simulink model "test_sys3"  (R2013b)
settings: Solver=ode45  StartTime=0.0  StopTime=5000  RelTol=1e-3
undefined symbols (not defined in the file or in its folder): twiddle_factors
libraries: xbsIndex_r4 x3475, casper_library_misc x231, xps_library x1
(part 1 of 38)
settings Model: Creator=root  LastModifiedBy=root

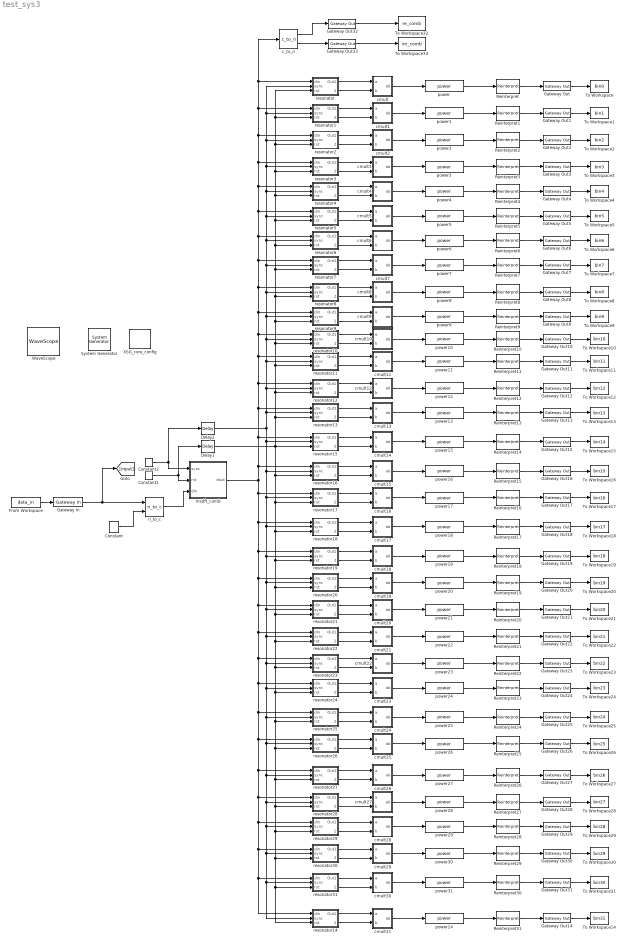
== system test_sys3 ==
  " System Generator" : xbsIndex_r4/ System Generator  Tag=genX  xilinxfamily=Kintex7  part=xc7k325t  speed=-3  package=fbg676  synthesis_tool=XST  clock_wrapper=Clock Enables  directory=./netlist  proj_type=Project Navigator  Synth_file=XST Defaults  Impl_file=ISE Defaults  testbench=off  simulink_period=1  sysclk_period=10  dcm_input_clock_period=10  incr_netlist=off  trim_vbits=Everywhere in SubSystem  dbl_ovrd=According to Block Masks  core_generation=According to Block Masks  run_coregen=off  deprecated_control=off  eval_field=0  block_type=sysgen
  Constant : xbsIndex_r4/Constant  const=0  gui_display_data_type=Fixed-point  arith_type=Signed (2's comp)  n_bits=10  bin_pt=9  preci_type=Single  exp_width=8  frac_width=24  explicit_period=on  period=1  equ=P=C  opselect=C  inp2=PCIN>>17  opr=+  inp1=P  carry=CIN  dbl_ovrd=off  block_type=constant
  Constant1 : xbsIndex_r4/Constant  const=0  gui_display_data_type=Boolean  arith_type=Boolean  n_bits=16  bin_pt=14  preci_type=Single  exp_width=8  frac_width=24  explicit_period=on  period=1  equ=P=C  opselect=C  inp2=PCIN>>17  opr=+  inp1=P  carry=CIN  dbl_ovrd=off  block_type=constant
  Constant2 : xbsIndex_r4/Constant  const=1  gui_display_data_type=Boolean  arith_type=Boolean  n_bits=16  bin_pt=14  preci_type=Single  exp_width=8  frac_width=24  explicit_period=on  period=1  equ=P=C  opselect=C  inp2=PCIN>>17  opr=+  inp1=P  carry=CIN  dbl_ovrd=off  block_type=constant
  Delay1 : xbsIndex_r4/Delay  rst=off  infoeditControl=Selection of Reset will increase slice count due to use of real FFs and instead of SRLs  en=off  latency=1  dbl_ovrd=off  reg_retiming=off  block_type=delay
  Delay2 : xbsIndex_r4/Delay  rst=off  infoeditControl=Selection of Reset will increase slice count due to use of real FFs and instead of SRLs  en=off  latency=1  dbl_ovrd=off  reg_retiming=off  block_type=delay
  From Workspace : FromWorkspace  VariableName=data_in  SampleTime=0
  Gateway In : xbsIndex_r4/Gateway In  gui_display_data_type=Fixed-point  arith_type="Signed  (2's comp)"  n_bits=10  bin_pt=9  preci_type=Single  exp_width=8  frac_width=24  quantization="Round  (unbiased: +/- Inf)"  overflow=Saturate  period=1  dbl_ovrd=off  timing_constraint=None  locs_specified=off  LOCs={}  UseAsADC=off  ADCChannel='1'  inherit_from_input=off  hdl_port=on  block_type=gatewayin
  Gateway Out{,1..33} (34 alike) : xbsIndex_r4/Gateway Out  inherit_from_input=off  hdl_port=on  timing_constraint=None  locs_specified=off  LOCs={}  UseAsDAC=off  DACChannel='1'  block_type=gatewayout
  Reinterpret{,1..31} (32 alike) : xbsIndex_r4/Reinterpret  force_arith_type=off  arith_type=Unsigned  force_bin_pt=on  bin_pt=0  block_type=reinterpret
  To Workspace : ToWorkspace  VariableName=bin0  SampleTime=-1  SaveFormat=Timeseries
  To Workspace1 : ToWorkspace  VariableName=bin1  SampleTime=-1  SaveFormat=Timeseries
  To Workspace10 : ToWorkspace  VariableName=bin10  SampleTime=-1  SaveFormat=Timeseries
  To Workspace11 : ToWorkspace  VariableName=bin11  SampleTime=-1  SaveFormat=Timeseries
  To Workspace12 : ToWorkspace  VariableName=bin12  SampleTime=-1  SaveFormat=Timeseries
  To Workspace13 : ToWorkspace  VariableName=bin13  SampleTime=-1  SaveFormat=Timeseries
  To Workspace14 : ToWorkspace  VariableName=bin31  SampleTime=-1  SaveFormat=Timeseries
  To Workspace15 : ToWorkspace  VariableName=bin14  SampleTime=-1  SaveFormat=Timeseries
  To Workspace16 : ToWorkspace  VariableName=bin15  SampleTime=-1  SaveFormat=Timeseries
  To Workspace17 : ToWorkspace  VariableName=bin16  SampleTime=-1  SaveFormat=Timeseries
  To Workspace18 : ToWorkspace  VariableName=bin17  SampleTime=-1  SaveFormat=Timeseries
  To Workspace19 : ToWorkspace  VariableName=bin18  SampleTime=-1  SaveFormat=Timeseries
  To Workspace2 : ToWorkspace  VariableName=bin2  SampleTime=-1  SaveFormat=Timeseries
  To Workspace20 : ToWorkspace  VariableName=bin19  SampleTime=-1  SaveFormat=Timeseries
  To Workspace21 : ToWorkspace  VariableName=bin20  SampleTime=-1  SaveFormat=Timeseries
  To Workspace22 : ToWorkspace  VariableName=bin21  SampleTime=-1  SaveFormat=Timeseries
  To Workspace23 : ToWorkspace  VariableName=bin22  SampleTime=-1  SaveFormat=Timeseries
  To Workspace24 : ToWorkspace  VariableName=bin23  SampleTime=-1  SaveFormat=Timeseries
  To Workspace25 : ToWorkspace  VariableName=bin24  SampleTime=-1  SaveFormat=Timeseries
  To Workspace26 : ToWorkspace  VariableName=bin25  SampleTime=-1  SaveFormat=Timeseries
  To Workspace27 : ToWorkspace  VariableName=bin26  SampleTime=-1  SaveFormat=Timeseries
  To Workspace28 : ToWorkspace  VariableName=bin27  SampleTime=-1  SaveFormat=Timeseries
  To Workspace29 : ToWorkspace  VariableName=bin28  SampleTime=-1  SaveFormat=Timeseries
  To Workspace3 : ToWorkspace  VariableName=bin3  SampleTime=-1  SaveFormat=Timeseries
  To Workspace30 : ToWorkspace  VariableName=bin29  SampleTime=-1  SaveFormat=Timeseries
  To Workspace31 : ToWorkspace  VariableName=bin30  SampleTime=-1  SaveFormat=Timeseries
  To Workspace32 : ToWorkspace  VariableName=re_comb  SampleTime=-1  SaveFormat=Timeseries
  To Workspace33 : ToWorkspace  VariableName=im_comb  SampleTime=-1  SaveFormat=Timeseries
  To Workspace4 : ToWorkspace  VariableName=bin4  SampleTime=-1  SaveFormat=Timeseries
  To Workspace5 : ToWorkspace  VariableName=bin5  SampleTime=-1  SaveFormat=Timeseries
  To Workspace6 : ToWorkspace  VariableName=bin6  SampleTime=-1  SaveFormat=Timeseries
  To Workspace7 : ToWorkspace  VariableName=bin7  SampleTime=-1  SaveFormat=Timeseries
  To Workspace8 : ToWorkspace  VariableName=bin8  SampleTime=-1  SaveFormat=Timeseries
  To Workspace9 : ToWorkspace  VariableName=bin9  SampleTime=-1  SaveFormat=Timeseries
  WaveScope : xbsIndex_r4/WaveScope  block_type=wavescope
  XSG_core_config : xps_library/XSG_core_config  Tag=xps:xsg  hw_sys=ROACH2:sx475t  clk_src=sys_clk  ROACH_clk_src=sys_clk  ROACH2_clk_src=sys_clk  MKDIG_clk_src=sys_clk  clk_rate=100  sample_period=1  synthesis_tool=XST
  c_to_ri : casper_library_misc/c_to_ri  n_bits=11  bin_pt=9
      settings: AttributesFormatString=11_9 r/i
  cmult : Subsystem  AncestorBlock=casper_library_multipliers/cmult  mask(cmult){n_bits_a=40, bin_pt_a=22, n_bits_b=15, bin_pt_b=13, n_bits_ab=56, bin_pt_ab=35, quantization=Truncate, overflow=Wrap, in_latency=0, mult_latency=3, add_latency=1, conv_latency=1, conjugated=off, async=off, pipelined_enable=on, multiplier_implementation=behavioral HDL}
      mask prompts: n_bits_a "Number of Bits 'a'"; bin_pt_a "Binary Point 'a'"; n_bits_b "Number of Bits 'b'"; bin_pt_b "Binary Point 'b'"; n_bits_ab "Number of Bits 'ab'"; bin_pt_ab "Binary Point 'ab'"; in_latency "Input latency"; mult_latency "Multiplier Latency"; add_latency "Adder Latency"; conv_latency "Convert latency"; conjugated "Conjugate"; async "asynchronous operation"; pipelined_enable "enable pipeline"; multiplier_implementation "Multiplier implementation"
      mask help:
      | Multiplies two complex numbers using 4 multipliers and 2 adders.
      | Conjugation is optional.
      mask init:
      | cmult_init(gcb, ...
      |     'n_bits_a',n_bits_a, ...
      |     'bin_pt_a',bin_pt_a, ...
      |     'n_bits_b',n_bits_b, ...
      |     'bin_pt_b',bin_pt_b, ...
      |     'n_bits_ab',n_bits_ab, ...
      |     'bin_pt_ab',bin_pt_ab, ...
      |     'quantization',quantization, ...
      |     'overflow', overflow, ...
      |     'in_latency', in_latency, ...
      |     'mult_latency', mult_latency, ...
      |     'add_latency', add_latency, ...
      |     'conv_latency', conv_latency, ...
      |     'conjugated', conjugated, ...
      |     'multiplier_implementation', multiplier_implementation, ...
      |     'async', async, ...
      |     'pipelined_enable', pipelined_enable);
      settings: AttributesFormatString=|
      | 40_22 * 15_13 ==> 56_35
      | Truncate, Wrap
      | Latency=0
      mask TypeOptions quantization: Truncate | Round  (unbiased: +/- Inf) | Round  (unbiased: Even Values)
      mask TypeOptions overflow: Wrap | Saturate | Flag as error
      mask TypeOptions multiplier_implementation: behavioral HDL | standard core | embedded multiplier core
  cmult1 : Subsystem  AncestorBlock=casper_library_multipliers/cmult  mask(cmult){n_bits_a=40, bin_pt_a=22, n_bits_b=15, bin_pt_b=13, n_bits_ab=56, bin_pt_ab=35, quantization=Truncate, overflow=Wrap, in_latency=0, mult_latency=3, add_latency=1, conv_latency=1, conjugated=off, async=off, pipelined_enable=on, multiplier_implementation=behavioral HDL}
      mask prompts: n_bits_a "Number of Bits 'a'"; bin_pt_a "Binary Point 'a'"; n_bits_b "Number of Bits 'b'"; bin_pt_b "Binary Point 'b'"; n_bits_ab "Number of Bits 'ab'"; bin_pt_ab "Binary Point 'ab'"; in_latency "Input latency"; mult_latency "Multiplier Latency"; add_latency "Adder Latency"; conv_latency "Convert latency"; conjugated "Conjugate"; async "asynchronous operation"; pipelined_enable "enable pipeline"; multiplier_implementation "Multiplier implementation"
      mask help:
      | Multiplies two complex numbers using 4 multipliers and 2 adders.
      | Conjugation is optional.
      mask init: same as test_sys3/cmult
      settings: AttributesFormatString=|
      | 40_22 * 15_13 ==> 56_35
      | Truncate, Wrap
      | Latency=0
      mask TypeOptions quantization: Truncate | Round  (unbiased: +/- Inf) | Round  (unbiased: Even Values)
      mask TypeOptions overflow: Wrap | Saturate | Flag as error
      mask TypeOptions multiplier_implementation: behavioral HDL | standard core | embedded multiplier core
  cmult10 : Subsystem  AncestorBlock=casper_library_multipliers/cmult  mask(cmult){n_bits_a=40, bin_pt_a=22, n_bits_b=15, bin_pt_b=13, n_bits_ab=56, bin_pt_ab=35, quantization=Truncate, overflow=Wrap, in_latency=0, mult_latency=3, add_latency=1, conv_latency=1, conjugated=off, async=off, pipelined_enable=on, multiplier_implementation=behavioral HDL}
      mask prompts: n_bits_a "Number of Bits 'a'"; bin_pt_a "Binary Point 'a'"; n_bits_b "Number of Bits 'b'"; bin_pt_b "Binary Point 'b'"; n_bits_ab "Number of Bits 'ab'"; bin_pt_ab "Binary Point 'ab'"; in_latency "Input latency"; mult_latency "Multiplier Latency"; add_latency "Adder Latency"; conv_latency "Convert latency"; conjugated "Conjugate"; async "asynchronous operation"; pipelined_enable "enable pipeline"; multiplier_implementation "Multiplier implementation"
      mask help:
      | Multiplies two complex numbers using 4 multipliers and 2 adders.
      | Conjugation is optional.
      mask init: same as test_sys3/cmult
      settings: AttributesFormatString=|
      | 40_22 * 15_13 ==> 56_35
      | Truncate, Wrap
      | Latency=0
      mask TypeOptions quantization: Truncate | Round  (unbiased: +/- Inf) | Round  (unbiased: Even Values)
      mask TypeOptions overflow: Wrap | Saturate | Flag as error
      mask TypeOptions multiplier_implementation: behavioral HDL | standard core | embedded multiplier core
  cmult11 : Subsystem  AncestorBlock=casper_library_multipliers/cmult  mask(cmult){n_bits_a=40, bin_pt_a=22, n_bits_b=15, bin_pt_b=13, n_bits_ab=56, bin_pt_ab=35, quantization=Truncate, overflow=Wrap, in_latency=0, mult_latency=3, add_latency=1, conv_latency=1, conjugated=off, async=off, pipelined_enable=on, multiplier_implementation=behavioral HDL}
      mask prompts: n_bits_a "Number of Bits 'a'"; bin_pt_a "Binary Point 'a'"; n_bits_b "Number of Bits 'b'"; bin_pt_b "Binary Point 'b'"; n_bits_ab "Number of Bits 'ab'"; bin_pt_ab "Binary Point 'ab'"; in_latency "Input latency"; mult_latency "Multiplier Latency"; add_latency "Adder Latency"; conv_latency "Convert latency"; conjugated "Conjugate"; async "asynchronous operation"; pipelined_enable "enable pipeline"; multiplier_implementation "Multiplier implementation"
      mask help:
      | Multiplies two complex numbers using 4 multipliers and 2 adders.
      | Conjugation is optional.
      mask init: same as test_sys3/cmult
      settings: AttributesFormatString=|
      | 40_22 * 15_13 ==> 56_35
      | Truncate, Wrap
      | Latency=0
      mask TypeOptions quantization: Truncate | Round  (unbiased: +/- Inf) | Round  (unbiased: Even Values)
      mask TypeOptions overflow: Wrap | Saturate | Flag as error
      mask TypeOptions multiplier_implementation: behavioral HDL | standard core | embedded multiplier core
  cmult12 : Subsystem  AncestorBlock=casper_library_multipliers/cmult  mask(cmult){n_bits_a=40, bin_pt_a=22, n_bits_b=15, bin_pt_b=13, n_bits_ab=56, bin_pt_ab=35, quantization=Truncate, overflow=Wrap, in_latency=0, mult_latency=3, add_latency=1, conv_latency=1, conjugated=off, async=off, pipelined_enable=on, multiplier_implementation=behavioral HDL}
      mask prompts: n_bits_a "Number of Bits 'a'"; bin_pt_a "Binary Point 'a'"; n_bits_b "Number of Bits 'b'"; bin_pt_b "Binary Point 'b'"; n_bits_ab "Number of Bits 'ab'"; bin_pt_ab "Binary Point 'ab'"; in_latency "Input latency"; mult_latency "Multiplier Latency"; add_latency "Adder Latency"; conv_latency "Convert latency"; conjugated "Conjugate"; async "asynchronous operation"; pipelined_enable "enable pipeline"; multiplier_implementation "Multiplier implementation"
      mask help:
      | Multiplies two complex numbers using 4 multipliers and 2 adders.
      | Conjugation is optional.
      mask init: same as test_sys3/cmult
      settings: AttributesFormatString=|
      | 40_22 * 15_13 ==> 56_35
      | Truncate, Wrap
      | Latency=0
      mask TypeOptions quantization: Truncate | Round  (unbiased: +/- Inf) | Round  (unbiased: Even Values)
      mask TypeOptions overflow: Wrap | Saturate | Flag as error
      mask TypeOptions multiplier_implementation: behavioral HDL | standard core | embedded multiplier core
  cmult13 : Subsystem  AncestorBlock=casper_library_multipliers/cmult  mask(cmult){n_bits_a=40, bin_pt_a=22, n_bits_b=15, bin_pt_b=13, n_bits_ab=56, bin_pt_ab=35, quantization=Truncate, overflow=Wrap, in_latency=0, mult_latency=3, add_latency=1, conv_latency=1, conjugated=off, async=off, pipelined_enable=on, multiplier_implementation=behavioral HDL}
      mask prompts: n_bits_a "Number of Bits 'a'"; bin_pt_a "Binary Point 'a'"; n_bits_b "Number of Bits 'b'"; bin_pt_b "Binary Point 'b'"; n_bits_ab "Number of Bits 'ab'"; bin_pt_ab "Binary Point 'ab'"; in_latency "Input latency"; mult_latency "Multiplier Latency"; add_latency "Adder Latency"; conv_latency "Convert latency"; conjugated "Conjugate"; async "asynchronous operation"; pipelined_enable "enable pipeline"; multiplier_implementation "Multiplier implementation"
      mask help:
      | Multiplies two complex numbers using 4 multipliers and 2 adders.
      | Conjugation is optional.
      mask init: same as test_sys3/cmult
      settings: AttributesFormatString=|
      | 40_22 * 15_13 ==> 56_35
      | Truncate, Wrap
      | Latency=0
      mask TypeOptions quantization: Truncate | Round  (unbiased: +/- Inf) | Round  (unbiased: Even Values)
      mask TypeOptions overflow: Wrap | Saturate | Flag as error
      mask TypeOptions multiplier_implementation: behavioral HDL | standard core | embedded multiplier core
  cmult14 : Subsystem  AncestorBlock=casper_library_multipliers/cmult  mask(cmult){n_bits_a=40, bin_pt_a=22, n_bits_b=15, bin_pt_b=13, n_bits_ab=56, bin_pt_ab=35, quantization=Truncate, overflow=Wrap, in_latency=0, mult_latency=3, add_latency=1, conv_latency=1, conjugated=off, async=off, pipelined_enable=on, multiplier_implementation=behavioral HDL}
      mask prompts: n_bits_a "Number of Bits 'a'"; bin_pt_a "Binary Point 'a'"; n_bits_b "Number of Bits 'b'"; bin_pt_b "Binary Point 'b'"; n_bits_ab "Number of Bits 'ab'"; bin_pt_ab "Binary Point 'ab'"; in_latency "Input latency"; mult_latency "Multiplier Latency"; add_latency "Adder Latency"; conv_latency "Convert latency"; conjugated "Conjugate"; async "asynchronous operation"; pipelined_enable "enable pipeline"; multiplier_implementation "Multiplier implementation"
      mask help:
      | Multiplies two complex numbers using 4 multipliers and 2 adders.
      | Conjugation is optional.
      mask init: same as test_sys3/cmult
      settings: AttributesFormatString=|
      | 40_22 * 15_13 ==> 56_35
      | Truncate, Wrap
      | Latency=0
      mask TypeOptions quantization: Truncate | Round  (unbiased: +/- Inf) | Round  (unbiased: Even Values)
      mask TypeOptions overflow: Wrap | Saturate | Flag as error
      mask TypeOptions multiplier_implementation: behavioral HDL | standard core | embedded multiplier core
  cmult15 : Subsystem  AncestorBlock=casper_library_multipliers/cmult  mask(cmult){n_bits_a=40, bin_pt_a=22, n_bits_b=15, bin_pt_b=13, n_bits_ab=56, bin_pt_ab=35, quantization=Truncate, overflow=Wrap, in_latency=0, mult_latency=3, add_latency=1, conv_latency=1, conjugated=off, async=off, pipelined_enable=on, multiplier_implementation=behavioral HDL}
      mask prompts: n_bits_a "Number of Bits 'a'"; bin_pt_a "Binary Point 'a'"; n_bits_b "Number of Bits 'b'"; bin_pt_b "Binary Point 'b'"; n_bits_ab "Number of Bits 'ab'"; bin_pt_ab "Binary Point 'ab'"; in_latency "Input latency"; mult_latency "Multiplier Latency"; add_latency "Adder Latency"; conv_latency "Convert latency"; conjugated "Conjugate"; async "asynchronous operation"; pipelined_enable "enable pipeline"; multiplier_implementation "Multiplier implementation"
      mask help:
      | Multiplies two complex numbers using 4 multipliers and 2 adders.
      | Conjugation is optional.
      mask init: same as test_sys3/cmult
      settings: AttributesFormatString=|
      | 40_22 * 15_13 ==> 56_35
      | Truncate, Wrap
      | Latency=0
      mask TypeOptions quantization: Truncate | Round  (unbiased: +/- Inf) | Round  (unbiased: Even Values)
      mask TypeOptions overflow: Wrap | Saturate | Flag as error
      mask TypeOptions multiplier_implementation: behavioral HDL | standard core | embedded multiplier core
  cmult16 : Subsystem  AncestorBlock=casper_library_multipliers/cmult  mask(cmult){n_bits_a=40, bin_pt_a=22, n_bits_b=15, bin_pt_b=13, n_bits_ab=56, bin_pt_ab=35, quantization=Truncate, overflow=Wrap, in_latency=0, mult_latency=3, add_latency=1, conv_latency=1, conjugated=off, async=off, pipelined_enable=on, multiplier_implementation=behavioral HDL}
      mask prompts: n_bits_a "Number of Bits 'a'"; bin_pt_a "Binary Point 'a'"; n_bits_b "Number of Bits 'b'"; bin_pt_b "Binary Point 'b'"; n_bits_ab "Number of Bits 'ab'"; bin_pt_ab "Binary Point 'ab'"; in_latency "Input latency"; mult_latency "Multiplier Latency"; add_latency "Adder Latency"; conv_latency "Convert latency"; conjugated "Conjugate"; async "asynchronous operation"; pipelined_enable "enable pipeline"; multiplier_implementation "Multiplier implementation"
      mask help:
      | Multiplies two complex numbers using 4 multipliers and 2 adders.
      | Conjugation is optional.
      mask init: same as test_sys3/cmult
      settings: AttributesFormatString=|
      | 40_22 * 15_13 ==> 56_35
      | Truncate, Wrap
      | Latency=0
      mask TypeOptions quantization: Truncate | Round  (unbiased: +/- Inf) | Round  (unbiased: Even Values)
      mask TypeOptions overflow: Wrap | Saturate | Flag as error
      mask TypeOptions multiplier_implementation: behavioral HDL | standard core | embedded multiplier core
  cmult17 : Subsystem  AncestorBlock=casper_library_multipliers/cmult  mask(cmult){n_bits_a=40, bin_pt_a=22, n_bits_b=15, bin_pt_b=13, n_bits_ab=56, bin_pt_ab=35, quantization=Truncate, overflow=Wrap, in_latency=0, mult_latency=3, add_latency=1, conv_latency=1, conjugated=off, async=off, pipelined_enable=on, multiplier_implementation=behavioral HDL}
      mask prompts: n_bits_a "Number of Bits 'a'"; bin_pt_a "Binary Point 'a'"; n_bits_b "Number of Bits 'b'"; bin_pt_b "Binary Point 'b'"; n_bits_ab "Number of Bits 'ab'"; bin_pt_ab "Binary Point 'ab'"; in_latency "Input latency"; mult_latency "Multiplier Latency"; add_latency "Adder Latency"; conv_latency "Convert latency"; conjugated "Conjugate"; async "asynchronous operation"; pipelined_enable "enable pipeline"; multiplier_implementation "Multiplier implementation"
      mask help:
      | Multiplies two complex numbers using 4 multipliers and 2 adders.
      | Conjugation is optional.
      mask init: same as test_sys3/cmult
      settings: AttributesFormatString=|
      | 40_22 * 15_13 ==> 56_35
      | Truncate, Wrap
      | Latency=0
      mask TypeOptions quantization: Truncate | Round  (unbiased: +/- Inf) | Round  (unbiased: Even Values)
      mask TypeOptions overflow: Wrap | Saturate | Flag as error
      mask TypeOptions multiplier_implementation: behavioral HDL | standard core | embedded multiplier core
  cmult18 : Subsystem  AncestorBlock=casper_library_multipliers/cmult  mask(cmult){n_bits_a=40, bin_pt_a=22, n_bits_b=15, bin_pt_b=13, n_bits_ab=56, bin_pt_ab=35, quantization=Truncate, overflow=Wrap, in_latency=0, mult_latency=3, add_latency=1, conv_latency=1, conjugated=off, async=off, pipelined_enable=on, multiplier_implementation=behavioral HDL}
      mask prompts: n_bits_a "Number of Bits 'a'"; bin_pt_a "Binary Point 'a'"; n_bits_b "Number of Bits 'b'"; bin_pt_b "Binary Point 'b'"; n_bits_ab "Number of Bits 'ab'"; bin_pt_ab "Binary Point 'ab'"; in_latency "Input latency"; mult_latency "Multiplier Latency"; add_latency "Adder Latency"; conv_latency "Convert latency"; conjugated "Conjugate"; async "asynchronous operation"; pipelined_enable "enable pipeline"; multiplier_implementation "Multiplier implementation"
      mask help:
      | Multiplies two complex numbers using 4 multipliers and 2 adders.
      | Conjugation is optional.
      mask init: same as test_sys3/cmult
      settings: AttributesFormatString=|
      | 40_22 * 15_13 ==> 56_35
      | Truncate, Wrap
      | Latency=0
      mask TypeOptions quantization: Truncate | Round  (unbiased: +/- Inf) | Round  (unbiased: Even Values)
      mask TypeOptions overflow: Wrap | Saturate | Flag as error
      mask TypeOptions multiplier_implementation: behavioral HDL | standard core | embedded multiplier core
  cmult19 : Subsystem  AncestorBlock=casper_library_multipliers/cmult  mask(cmult){n_bits_a=40, bin_pt_a=22, n_bits_b=15, bin_pt_b=13, n_bits_ab=56, bin_pt_ab=35, quantization=Truncate, overflow=Wrap, in_latency=0, mult_latency=3, add_latency=1, conv_latency=1, conjugated=off, async=off, pipelined_enable=on, multiplier_implementation=behavioral HDL}
      mask prompts: n_bits_a "Number of Bits 'a'"; bin_pt_a "Binary Point 'a'"; n_bits_b "Number of Bits 'b'"; bin_pt_b "Binary Point 'b'"; n_bits_ab "Number of Bits 'ab'"; bin_pt_ab "Binary Point 'ab'"; in_latency "Input latency"; mult_latency "Multiplier Latency"; add_latency "Adder Latency"; conv_latency "Convert latency"; conjugated "Conjugate"; async "asynchronous operation"; pipelined_enable "enable pipeline"; multiplier_implementation "Multiplier implementation"
      mask help:
      | Multiplies two complex numbers using 4 multipliers and 2 adders.
      | Conjugation is optional.
      mask init: same as test_sys3/cmult
      settings: AttributesFormatString=|
      | 40_22 * 15_13 ==> 56_35
      | Truncate, Wrap
      | Latency=0
      mask TypeOptions quantization: Truncate | Round  (unbiased: +/- Inf) | Round  (unbiased: Even Values)
      mask TypeOptions overflow: Wrap | Saturate | Flag as error
      mask TypeOptions multiplier_implementation: behavioral HDL | standard core | embedded multiplier core
  cmult2 : Subsystem  AncestorBlock=casper_library_multipliers/cmult  mask(cmult){n_bits_a=40, bin_pt_a=22, n_bits_b=15, bin_pt_b=13, n_bits_ab=56, bin_pt_ab=35, quantization=Truncate, overflow=Wrap, in_latency=0, mult_latency=3, add_latency=1, conv_latency=1, conjugated=off, async=off, pipelined_enable=on, multiplier_implementation=behavioral HDL}
      mask prompts: n_bits_a "Number of Bits 'a'"; bin_pt_a "Binary Point 'a'"; n_bits_b "Number of Bits 'b'"; bin_pt_b "Binary Point 'b'"; n_bits_ab "Number of Bits 'ab'"; bin_pt_ab "Binary Point 'ab'"; in_latency "Input latency"; mult_latency "Multiplier Latency"; add_latency "Adder Latency"; conv_latency "Convert latency"; conjugated "Conjugate"; async "asynchronous operation"; pipelined_enable "enable pipeline"; multiplier_implementation "Multiplier implementation"
      mask help:
      | Multiplies two complex numbers using 4 multipliers and 2 adders.
      | Conjugation is optional.
      mask init: same as test_sys3/cmult
      settings: AttributesFormatString=|
      | 40_22 * 15_13 ==> 56_35
      | Truncate, Wrap
      | Latency=0
      mask TypeOptions quantization: Truncate | Round  (unbiased: +/- Inf) | Round  (unbiased: Even Values)
      mask TypeOptions overflow: Wrap | Saturate | Flag as error
      mask TypeOptions multiplier_implementation: behavioral HDL | standard core | embedded multiplier core
  cmult20 : Subsystem  AncestorBlock=casper_library_multipliers/cmult  mask(cmult){n_bits_a=40, bin_pt_a=22, n_bits_b=15, bin_pt_b=13, n_bits_ab=56, bin_pt_ab=35, quantization=Truncate, overflow=Wrap, in_latency=0, mult_latency=3, add_latency=1, conv_latency=1, conjugated=off, async=off, pipelined_enable=on, multiplier_implementation=behavioral HDL}
      mask prompts: n_bits_a "Number of Bits 'a'"; bin_pt_a "Binary Point 'a'"; n_bits_b "Number of Bits 'b'"; bin_pt_b "Binary Point 'b'"; n_bits_ab "Number of Bits 'ab'"; bin_pt_ab "Binary Point 'ab'"; in_latency "Input latency"; mult_latency "Multiplier Latency"; add_latency "Adder Latency"; conv_latency "Convert latency"; conjugated "Conjugate"; async "asynchronous operation"; pipelined_enable "enable pipeline"; multiplier_implementation "Multiplier implementation"
      mask help:
      | Multiplies two complex numbers using 4 multipliers and 2 adders.
      | Conjugation is optional.
      mask init: same as test_sys3/cmult
      settings: AttributesFormatString=|
      | 40_22 * 15_13 ==> 56_35
      | Truncate, Wrap
      | Latency=0
      mask TypeOptions quantization: Truncate | Round  (unbiased: +/- Inf) | Round  (unbiased: Even Values)
      mask TypeOptions overflow: Wrap | Saturate | Flag as error
      mask TypeOptions multiplier_implementation: behavioral HDL | standard core | embedded multiplier core
  cmult21 : Subsystem  AncestorBlock=casper_library_multipliers/cmult  mask(cmult){n_bits_a=40, bin_pt_a=22, n_bits_b=15, bin_pt_b=13, n_bits_ab=56, bin_pt_ab=35, quantization=Truncate, overflow=Wrap, in_latency=0, mult_latency=3, add_latency=1, conv_latency=1, conjugated=off, async=off, pipelined_enable=on, multiplier_implementation=behavioral HDL}
      mask prompts: n_bits_a "Number of Bits 'a'"; bin_pt_a "Binary Point 'a'"; n_bits_b "Number of Bits 'b'"; bin_pt_b "Binary Point 'b'"; n_bits_ab "Number of Bits 'ab'"; bin_pt_ab "Binary Point 'ab'"; in_latency "Input latency"; mult_latency "Multiplier Latency"; add_latency "Adder Latency"; conv_latency "Convert latency"; conjugated "Conjugate"; async "asynchronous operation"; pipelined_enable "enable pipeline"; multiplier_implementation "Multiplier implementation"
      mask help:
      | Multiplies two complex numbers using 4 multipliers and 2 adders.
      | Conjugation is optional.
      mask init: same as test_sys3/cmult
      settings: AttributesFormatString=|
      | 40_22 * 15_13 ==> 56_35
      | Truncate, Wrap
      | Latency=0
      mask TypeOptions quantization: Truncate | Round  (unbiased: +/- Inf) | Round  (unbiased: Even Values)
      mask TypeOptions overflow: Wrap | Saturate | Flag as error
      mask TypeOptions multiplier_implementation: behavioral HDL | standard core | embedded multiplier core
  cmult22 : Subsystem  AncestorBlock=casper_library_multipliers/cmult  mask(cmult){n_bits_a=40, bin_pt_a=22, n_bits_b=15, bin_pt_b=13, n_bits_ab=56, bin_pt_ab=35, quantization=Truncate, overflow=Wrap, in_latency=0, mult_latency=3, add_latency=1, conv_latency=1, conjugated=off, async=off, pipelined_enable=on, multiplier_implementation=behavioral HDL}
      mask prompts: n_bits_a "Number of Bits 'a'"; bin_pt_a "Binary Point 'a'"; n_bits_b "Number of Bits 'b'"; bin_pt_b "Binary Point 'b'"; n_bits_ab "Number of Bits 'ab'"; bin_pt_ab "Binary Point 'ab'"; in_latency "Input latency"; mult_latency "Multiplier Latency"; add_latency "Adder Latency"; conv_latency "Convert latency"; conjugated "Conjugate"; async "asynchronous operation"; pipelined_enable "enable pipeline"; multiplier_implementation "Multiplier implementation"
      mask help:
      | Multiplies two complex numbers using 4 multipliers and 2 adders.
      | Conjugation is optional.
      mask init: same as test_sys3/cmult
      settings: AttributesFormatString=|
      | 40_22 * 15_13 ==> 56_35
      | Truncate, Wrap
      | Latency=0
      mask TypeOptions quantization: Truncate | Round  (unbiased: +/- Inf) | Round  (unbiased: Even Values)
      mask TypeOptions overflow: Wrap | Saturate | Flag as error
      mask TypeOptions multiplier_implementation: behavioral HDL | standard core | embedded multiplier core
  cmult23 : Subsystem  AncestorBlock=casper_library_multipliers/cmult  mask(cmult){n_bits_a=40, bin_pt_a=22, n_bits_b=15, bin_pt_b=13, n_bits_ab=56, bin_pt_ab=35, quantization=Truncate, overflow=Wrap, in_latency=0, mult_latency=3, add_latency=1, conv_latency=1, conjugated=off, async=off, pipelined_enable=on, multiplier_implementation=behavioral HDL}
      mask prompts: n_bits_a "Number of Bits 'a'"; bin_pt_a "Binary Point 'a'"; n_bits_b "Number of Bits 'b'"; bin_pt_b "Binary Point 'b'"; n_bits_ab "Number of Bits 'ab'"; bin_pt_ab "Binary Point 'ab'"; in_latency "Input latency"; mult_latency "Multiplier Latency"; add_latency "Adder Latency"; conv_latency "Convert latency"; conjugated "Conjugate"; async "asynchronous operation"; pipelined_enable "enable pipeline"; multiplier_implementation "Multiplier implementation"
      mask help:
      | Multiplies two complex numbers using 4 multipliers and 2 adders.
      | Conjugation is optional.
      mask init: same as test_sys3/cmult
      settings: AttributesFormatString=|
      | 40_22 * 15_13 ==> 56_35
      | Truncate, Wrap
      | Latency=0
      mask TypeOptions quantization: Truncate | Round  (unbiased: +/- Inf) | Round  (unbiased: Even Values)
      mask TypeOptions overflow: Wrap | Saturate | Flag as error
      mask TypeOptions multiplier_implementation: behavioral HDL | standard core | embedded multiplier core
  cmult24 : Subsystem  AncestorBlock=casper_library_multipliers/cmult  mask(cmult){n_bits_a=40, bin_pt_a=22, n_bits_b=15, bin_pt_b=13, n_bits_ab=56, bin_pt_ab=35, quantization=Truncate, overflow=Wrap, in_latency=0, mult_latency=3, add_latency=1, conv_latency=1, conjugated=off, async=off, pipelined_enable=on, multiplier_implementation=behavioral HDL}
      mask prompts: n_bits_a "Number of Bits 'a'"; bin_pt_a "Binary Point 'a'"; n_bits_b "Number of Bits 'b'"; bin_pt_b "Binary Point 'b'"; n_bits_ab "Number of Bits 'ab'"; bin_pt_ab "Binary Point 'ab'"; in_latency "Input latency"; mult_latency "Multiplier Latency"; add_latency "Adder Latency"; conv_latency "Convert latency"; conjugated "Conjugate"; async "asynchronous operation"; pipelined_enable "enable pipeline"; multiplier_implementation "Multiplier implementation"
      mask help:
      | Multiplies two complex numbers using 4 multipliers and 2 adders.
      | Conjugation is optional.
      mask init: same as test_sys3/cmult
      settings: AttributesFormatString=|
      | 40_22 * 15_13 ==> 56_35
      | Truncate, Wrap
      | Latency=0
      mask TypeOptions quantization: Truncate | Round  (unbiased: +/- Inf) | Round  (unbiased: Even Values)
      mask TypeOptions overflow: Wrap | Saturate | Flag as error
      mask TypeOptions multiplier_implementation: behavioral HDL | standard core | embedded multiplier core
  cmult25 : Subsystem  AncestorBlock=casper_library_multipliers/cmult  mask(cmult){n_bits_a=40, bin_pt_a=22, n_bits_b=15, bin_pt_b=13, n_bits_ab=56, bin_pt_ab=35, quantization=Truncate, overflow=Wrap, in_latency=0, mult_latency=3, add_latency=1, conv_latency=1, conjugated=off, async=off, pipelined_enable=on, multiplier_implementation=behavioral HDL}
      mask prompts: n_bits_a "Number of Bits 'a'"; bin_pt_a "Binary Point 'a'"; n_bits_b "Number of Bits 'b'"; bin_pt_b "Binary Point 'b'"; n_bits_ab "Number of Bits 'ab'"; bin_pt_ab "Binary Point 'ab'"; in_latency "Input latency"; mult_latency "Multiplier Latency"; add_latency "Adder Latency"; conv_latency "Convert latency"; conjugated "Conjugate"; async "asynchronous operation"; pipelined_enable "enable pipeline"; multiplier_implementation "Multiplier implementation"
      mask help:
      | Multiplies two complex numbers using 4 multipliers and 2 adders.
      | Conjugation is optional.
      mask init: same as test_sys3/cmult
      settings: AttributesFormatString=|
      | 40_22 * 15_13 ==> 56_35
      | Truncate, Wrap
      | Latency=0
      mask TypeOptions quantization: Truncate | Round  (unbiased: +/- Inf) | Round  (unbiased: Even Values)
      mask TypeOptions overflow: Wrap | Saturate | Flag as error
      mask TypeOptions multiplier_implementation: behavioral HDL | standard core | embedded multiplier core
  cmult26 : Subsystem  AncestorBlock=casper_library_multipliers/cmult  mask(cmult){n_bits_a=40, bin_pt_a=22, n_bits_b=15, bin_pt_b=13, n_bits_ab=56, bin_pt_ab=35, quantization=Truncate, overflow=Wrap, in_latency=0, mult_latency=3, add_latency=1, conv_latency=1, conjugated=off, async=off, pipelined_enable=on, multiplier_implementation=behavioral HDL}
      mask prompts: n_bits_a "Number of Bits 'a'"; bin_pt_a "Binary Point 'a'"; n_bits_b "Number of Bits 'b'"; bin_pt_b "Binary Point 'b'"; n_bits_ab "Number of Bits 'ab'"; bin_pt_ab "Binary Point 'ab'"; in_latency "Input latency"; mult_latency "Multiplier Latency"; add_latency "Adder Latency"; conv_latency "Convert latency"; conjugated "Conjugate"; async "asynchronous operation"; pipelined_enable "enable pipeline"; multiplier_implementation "Multiplier implementation"
      mask help:
      | Multiplies two complex numbers using 4 multipliers and 2 adders.
      | Conjugation is optional.
      mask init: same as test_sys3/cmult
      settings: AttributesFormatString=|
      | 40_22 * 15_13 ==> 56_35
      | Truncate, Wrap
      | Latency=0
      mask TypeOptions quantization: Truncate | Round  (unbiased: +/- Inf) | Round  (unbiased: Even Values)
      mask TypeOptions overflow: Wrap | Saturate | Flag as error
      mask TypeOptions multiplier_implementation: behavioral HDL | standard core | embedded multiplier core
  cmult27 : Subsystem  AncestorBlock=casper_library_multipliers/cmult  mask(cmult){n_bits_a=40, bin_pt_a=22, n_bits_b=15, bin_pt_b=13, n_bits_ab=56, bin_pt_ab=35, quantization=Truncate, overflow=Wrap, in_latency=0, mult_latency=3, add_latency=1, conv_latency=1, conjugated=off, async=off, pipelined_enable=on, multiplier_implementation=behavioral HDL}
      mask prompts: n_bits_a "Number of Bits 'a'"; bin_pt_a "Binary Point 'a'"; n_bits_b "Number of Bits 'b'"; bin_pt_b "Binary Point 'b'"; n_bits_ab "Number of Bits 'ab'"; bin_pt_ab "Binary Point 'ab'"; in_latency "Input latency"; mult_latency "Multiplier Latency"; add_latency "Adder Latency"; conv_latency "Convert latency"; conjugated "Conjugate"; async "asynchronous operation"; pipelined_enable "enable pipeline"; multiplier_implementation "Multiplier implementation"
      mask help:
      | Multiplies two complex numbers using 4 multipliers and 2 adders.
      | Conjugation is optional.
      mask init: same as test_sys3/cmult
      settings: AttributesFormatString=|
      | 40_22 * 15_13 ==> 56_35
      | Truncate, Wrap
      | Latency=0
      mask TypeOptions quantization: Truncate | Round  (unbiased: +/- Inf) | Round  (unbiased: Even Values)
      mask TypeOptions overflow: Wrap | Saturate | Flag as error
      mask TypeOptions multiplier_implementation: behavioral HDL | standard core | embedded multiplier core
  cmult28 : Subsystem  AncestorBlock=casper_library_multipliers/cmult  mask(cmult){n_bits_a=40, bin_pt_a=22, n_bits_b=15, bin_pt_b=13, n_bits_ab=56, bin_pt_ab=35, quantization=Truncate, overflow=Wrap, in_latency=0, mult_latency=3, add_latency=1, conv_latency=1, conjugated=off, async=off, pipelined_enable=on, multiplier_implementation=behavioral HDL}
      mask prompts: n_bits_a "Number of Bits 'a'"; bin_pt_a "Binary Point 'a'"; n_bits_b "Number of Bits 'b'"; bin_pt_b "Binary Point 'b'"; n_bits_ab "Number of Bits 'ab'"; bin_pt_ab "Binary Point 'ab'"; in_latency "Input latency"; mult_latency "Multiplier Latency"; add_latency "Adder Latency"; conv_latency "Convert latency"; conjugated "Conjugate"; async "asynchronous operation"; pipelined_enable "enable pipeline"; multiplier_implementation "Multiplier implementation"
      mask help:
      | Multiplies two complex numbers using 4 multipliers and 2 adders.
      | Conjugation is optional.
      mask init: same as test_sys3/cmult
      settings: AttributesFormatString=|
      | 40_22 * 15_13 ==> 56_35
      | Truncate, Wrap
      | Latency=0
      mask TypeOptions quantization: Truncate | Round  (unbiased: +/- Inf) | Round  (unbiased: Even Values)
      mask TypeOptions overflow: Wrap | Saturate | Flag as error
      mask TypeOptions multiplier_implementation: behavioral HDL | standard core | embedded multiplier core
  cmult29 : Subsystem  AncestorBlock=casper_library_multipliers/cmult  mask(cmult){n_bits_a=40, bin_pt_a=22, n_bits_b=15, bin_pt_b=13, n_bits_ab=56, bin_pt_ab=35, quantization=Truncate, overflow=Wrap, in_latency=0, mult_latency=3, add_latency=1, conv_latency=1, conjugated=off, async=off, pipelined_enable=on, multiplier_implementation=behavioral HDL}
      mask prompts: n_bits_a "Number of Bits 'a'"; bin_pt_a "Binary Point 'a'"; n_bits_b "Number of Bits 'b'"; bin_pt_b "Binary Point 'b'"; n_bits_ab "Number of Bits 'ab'"; bin_pt_ab "Binary Point 'ab'"; in_latency "Input latency"; mult_latency "Multiplier Latency"; add_latency "Adder Latency"; conv_latency "Convert latency"; conjugated "Conjugate"; async "asynchronous operation"; pipelined_enable "enable pipeline"; multiplier_implementation "Multiplier implementation"
      mask help:
      | Multiplies two complex numbers using 4 multipliers and 2 adders.
      | Conjugation is optional.
      mask init: same as test_sys3/cmult
      settings: AttributesFormatString=|
      | 40_22 * 15_13 ==> 56_35
      | Truncate, Wrap
      | Latency=0
      mask TypeOptions quantization: Truncate | Round  (unbiased: +/- Inf) | Round  (unbiased: Even Values)
      mask TypeOptions overflow: Wrap | Saturate | Flag as error
      mask TypeOptions multiplier_implementation: behavioral HDL | standard core | embedded multiplier core
  cmult3 : Subsystem  AncestorBlock=casper_library_multipliers/cmult  mask(cmult){n_bits_a=40, bin_pt_a=22, n_bits_b=15, bin_pt_b=13, n_bits_ab=56, bin_pt_ab=35, quantization=Truncate, overflow=Wrap, in_latency=0, mult_latency=3, add_latency=1, conv_latency=1, conjugated=off, async=off, pipelined_enable=on, multiplier_implementation=behavioral HDL}
      mask prompts: n_bits_a "Number of Bits 'a'"; bin_pt_a "Binary Point 'a'"; n_bits_b "Number of Bits 'b'"; bin_pt_b "Binary Point 'b'"; n_bits_ab "Number of Bits 'ab'"; bin_pt_ab "Binary Point 'ab'"; in_latency "Input latency"; mult_latency "Multiplier Latency"; add_latency "Adder Latency"; conv_latency "Convert latency"; conjugated "Conjugate"; async "asynchronous operation"; pipelined_enable "enable pipeline"; multiplier_implementation "Multiplier implementation"
      mask help:
      | Multiplies two complex numbers using 4 multipliers and 2 adders.
      | Conjugation is optional.
      mask init: same as test_sys3/cmult
      settings: AttributesFormatString=|
      | 40_22 * 15_13 ==> 56_35
      | Truncate, Wrap
      | Latency=0
      mask TypeOptions quantization: Truncate | Round  (unbiased: +/- Inf) | Round  (unbiased: Even Values)
      mask TypeOptions overflow: Wrap | Saturate | Flag as error
      mask TypeOptions multiplier_implementation: behavioral HDL | standard core | embedded multiplier core
  cmult30 : Subsystem  AncestorBlock=casper_library_multipliers/cmult  mask(cmult){n_bits_a=40, bin_pt_a=22, n_bits_b=15, bin_pt_b=13, n_bits_ab=56, bin_pt_ab=35, quantization=Truncate, overflow=Wrap, in_latency=0, mult_latency=3, add_latency=1, conv_latency=1, conjugated=off, async=off, pipelined_enable=on, multiplier_implementation=behavioral HDL}
      mask prompts: n_bits_a "Number of Bits 'a'"; bin_pt_a "Binary Point 'a'"; n_bits_b "Number of Bits 'b'"; bin_pt_b "Binary Point 'b'"; n_bits_ab "Number of Bits 'ab'"; bin_pt_ab "Binary Point 'ab'"; in_latency "Input latency"; mult_latency "Multiplier Latency"; add_latency "Adder Latency"; conv_latency "Convert latency"; conjugated "Conjugate"; async "asynchronous operation"; pipelined_enable "enable pipeline"; multiplier_implementation "Multiplier implementation"
      mask help:
      | Multiplies two complex numbers using 4 multipliers and 2 adders.
      | Conjugation is optional.
      mask init: same as test_sys3/cmult
      settings: AttributesFormatString=|
      | 40_22 * 15_13 ==> 56_35
      | Truncate, Wrap
      | Latency=0
      mask TypeOptions quantization: Truncate | Round  (unbiased: +/- Inf) | Round  (unbiased: Even Values)
      mask TypeOptions overflow: Wrap | Saturate | Flag as error
      mask TypeOptions multiplier_implementation: behavioral HDL | standard core | embedded multiplier core
  cmult31 : Subsystem  AncestorBlock=casper_library_multipliers/cmult  mask(cmult){n_bits_a=40, bin_pt_a=22, n_bits_b=15, bin_pt_b=13, n_bits_ab=56, bin_pt_ab=35, quantization=Truncate, overflow=Wrap, in_latency=0, mult_latency=3, add_latency=1, conv_latency=1, conjugated=off, async=off, pipelined_enable=on, multiplier_implementation=behavioral HDL}
      mask prompts: n_bits_a "Number of Bits 'a'"; bin_pt_a "Binary Point 'a'"; n_bits_b "Number of Bits 'b'"; bin_pt_b "Binary Point 'b'"; n_bits_ab "Number of Bits 'ab'"; bin_pt_ab "Binary Point 'ab'"; in_latency "Input latency"; mult_latency "Multiplier Latency"; add_latency "Adder Latency"; conv_latency "Convert latency"; conjugated "Conjugate"; async "asynchronous operation"; pipelined_enable "enable pipeline"; multiplier_implementation "Multiplier implementation"
      mask help:
      | Multiplies two complex numbers using 4 multipliers and 2 adders.
      | Conjugation is optional.
      mask init: same as test_sys3/cmult
      settings: AttributesFormatString=|
      | 40_22 * 15_13 ==> 56_35
      | Truncate, Wrap
      | Latency=0
      mask TypeOptions quantization: Truncate | Round  (unbiased: +/- Inf) | Round  (unbiased: Even Values)
      mask TypeOptions overflow: Wrap | Saturate | Flag as error
      mask TypeOptions multiplier_implementation: behavioral HDL | standard core | embedded multiplier core
  cmult4 : Subsystem  AncestorBlock=casper_library_multipliers/cmult  mask(cmult){n_bits_a=40, bin_pt_a=22, n_bits_b=15, bin_pt_b=13, n_bits_ab=56, bin_pt_ab=35, quantization=Truncate, overflow=Wrap, in_latency=0, mult_latency=3, add_latency=1, conv_latency=1, conjugated=off, async=off, pipelined_enable=on, multiplier_implementation=behavioral HDL}
      mask prompts: n_bits_a "Number of Bits 'a'"; bin_pt_a "Binary Point 'a'"; n_bits_b "Number of Bits 'b'"; bin_pt_b "Binary Point 'b'"; n_bits_ab "Number of Bits 'ab'"; bin_pt_ab "Binary Point 'ab'"; in_latency "Input latency"; mult_latency "Multiplier Latency"; add_latency "Adder Latency"; conv_latency "Convert latency"; conjugated "Conjugate"; async "asynchronous operation"; pipelined_enable "enable pipeline"; multiplier_implementation "Multiplier implementation"
      mask help:
      | Multiplies two complex numbers using 4 multipliers and 2 adders.
      | Conjugation is optional.
      mask init: same as test_sys3/cmult
      settings: AttributesFormatString=|
      | 40_22 * 15_13 ==> 56_35
      | Truncate, Wrap
      | Latency=0
      mask TypeOptions quantization: Truncate | Round  (unbiased: +/- Inf) | Round  (unbiased: Even Values)
      mask TypeOptions overflow: Wrap | Saturate | Flag as error
      mask TypeOptions multiplier_implementation: behavioral HDL | standard core | embedded multiplier core
  cmult5 : Subsystem  AncestorBlock=casper_library_multipliers/cmult  mask(cmult){n_bits_a=40, bin_pt_a=22, n_bits_b=15, bin_pt_b=13, n_bits_ab=56, bin_pt_ab=35, quantization=Truncate, overflow=Wrap, in_latency=0, mult_latency=3, add_latency=1, conv_latency=1, conjugated=off, async=off, pipelined_enable=on, multiplier_implementation=behavioral HDL}
      mask prompts: n_bits_a "Number of Bits 'a'"; bin_pt_a "Binary Point 'a'"; n_bits_b "Number of Bits 'b'"; bin_pt_b "Binary Point 'b'"; n_bits_ab "Number of Bits 'ab'"; bin_pt_ab "Binary Point 'ab'"; in_latency "Input latency"; mult_latency "Multiplier Latency"; add_latency "Adder Latency"; conv_latency "Convert latency"; conjugated "Conjugate"; async "asynchronous operation"; pipelined_enable "enable pipeline"; multiplier_implementation "Multiplier implementation"
      mask help:
      | Multiplies two complex numbers using 4 multipliers and 2 adders.
      | Conjugation is optional.
      mask init: same as test_sys3/cmult
      settings: AttributesFormatString=|
      | 40_22 * 15_13 ==> 56_35
      | Truncate, Wrap
      | Latency=0
      mask TypeOptions quantization: Truncate | Round  (unbiased: +/- Inf) | Round  (unbiased: Even Values)
      mask TypeOptions overflow: Wrap | Saturate | Flag as error
      mask TypeOptions multiplier_implementation: behavioral HDL | standard core | embedded multiplier core
  cmult6 : Subsystem  AncestorBlock=casper_library_multipliers/cmult  mask(cmult){n_bits_a=40, bin_pt_a=22, n_bits_b=15, bin_pt_b=13, n_bits_ab=56, bin_pt_ab=35, quantization=Truncate, overflow=Wrap, in_latency=0, mult_latency=3, add_latency=1, conv_latency=1, conjugated=off, async=off, pipelined_enable=on, multiplier_implementation=behavioral HDL}
      mask prompts: n_bits_a "Number of Bits 'a'"; bin_pt_a "Binary Point 'a'"; n_bits_b "Number of Bits 'b'"; bin_pt_b "Binary Point 'b'"; n_bits_ab "Number of Bits 'ab'"; bin_pt_ab "Binary Point 'ab'"; in_latency "Input latency"; mult_latency "Multiplier Latency"; add_latency "Adder Latency"; conv_latency "Convert latency"; conjugated "Conjugate"; async "asynchronous operation"; pipelined_enable "enable pipeline"; multiplier_implementation "Multiplier implementation"
      mask help:
      | Multiplies two complex numbers using 4 multipliers and 2 adders.
      | Conjugation is optional.
      mask init: same as test_sys3/cmult
      settings: AttributesFormatString=|
      | 40_22 * 15_13 ==> 56_35
      | Truncate, Wrap
      | Latency=0
      mask TypeOptions quantization: Truncate | Round  (unbiased: +/- Inf) | Round  (unbiased: Even Values)
      mask TypeOptions overflow: Wrap | Saturate | Flag as error
      mask TypeOptions multiplier_implementation: behavioral HDL | standard core | embedded multiplier core
  cmult7 : Subsystem  AncestorBlock=casper_library_multipliers/cmult  mask(cmult){n_bits_a=40, bin_pt_a=22, n_bits_b=15, bin_pt_b=13, n_bits_ab=56, bin_pt_ab=35, quantization=Truncate, overflow=Wrap, in_latency=0, mult_latency=3, add_latency=1, conv_latency=1, conjugated=off, async=off, pipelined_enable=on, multiplier_implementation=behavioral HDL}
      mask prompts: n_bits_a "Number of Bits 'a'"; bin_pt_a "Binary Point 'a'"; n_bits_b "Number of Bits 'b'"; bin_pt_b "Binary Point 'b'"; n_bits_ab "Number of Bits 'ab'"; bin_pt_ab "Binary Point 'ab'"; in_latency "Input latency"; mult_latency "Multiplier Latency"; add_latency "Adder Latency"; conv_latency "Convert latency"; conjugated "Conjugate"; async "asynchronous operation"; pipelined_enable "enable pipeline"; multiplier_implementation "Multiplier implementation"
      mask help:
      | Multiplies two complex numbers using 4 multipliers and 2 adders.
      | Conjugation is optional.
      mask init: same as test_sys3/cmult
      settings: AttributesFormatString=|
      | 40_22 * 15_13 ==> 56_35
      | Truncate, Wrap
      | Latency=0
      mask TypeOptions quantization: Truncate | Round  (unbiased: +/- Inf) | Round  (unbiased: Even Values)
      mask TypeOptions overflow: Wrap | Saturate | Flag as error
      mask TypeOptions multiplier_implementation: behavioral HDL | standard core | embedded multiplier core
  cmult8 : Subsystem  AncestorBlock=casper_library_multipliers/cmult  mask(cmult){n_bits_a=40, bin_pt_a=22, n_bits_b=15, bin_pt_b=13, n_bits_ab=56, bin_pt_ab=35, quantization=Truncate, overflow=Wrap, in_latency=0, mult_latency=3, add_latency=1, conv_latency=1, conjugated=off, async=off, pipelined_enable=on, multiplier_implementation=behavioral HDL}
      mask prompts: n_bits_a "Number of Bits 'a'"; bin_pt_a "Binary Point 'a'"; n_bits_b "Number of Bits 'b'"; bin_pt_b "Binary Point 'b'"; n_bits_ab "Number of Bits 'ab'"; bin_pt_ab "Binary Point 'ab'"; in_latency "Input latency"; mult_latency "Multiplier Latency"; add_latency "Adder Latency"; conv_latency "Convert latency"; conjugated "Conjugate"; async "asynchronous operation"; pipelined_enable "enable pipeline"; multiplier_implementation "Multiplier implementation"
      mask help:
      | Multiplies two complex numbers using 4 multipliers and 2 adders.
      | Conjugation is optional.
      mask init: same as test_sys3/cmult
      settings: AttributesFormatString=|
      | 40_22 * 15_13 ==> 56_35
      | Truncate, Wrap
      | Latency=0
      mask TypeOptions quantization: Truncate | Round  (unbiased: +/- Inf) | Round  (unbiased: Even Values)
      mask TypeOptions overflow: Wrap | Saturate | Flag as error
      mask TypeOptions multiplier_implementation: behavioral HDL | standard core | embedded multiplier core
  cmult9 : Subsystem  AncestorBlock=casper_library_multipliers/cmult  mask(cmult){n_bits_a=40, bin_pt_a=22, n_bits_b=15, bin_pt_b=13, n_bits_ab=56, bin_pt_ab=35, quantization=Truncate, overflow=Wrap, in_latency=0, mult_latency=3, add_latency=1, conv_latency=1, conjugated=off, async=off, pipelined_enable=on, multiplier_implementation=behavioral HDL}
      mask prompts: n_bits_a "Number of Bits 'a'"; bin_pt_a "Binary Point 'a'"; n_bits_b "Number of Bits 'b'"; bin_pt_b "Binary Point 'b'"; n_bits_ab "Number of Bits 'ab'"; bin_pt_ab "Binary Point 'ab'"; in_latency "Input latency"; mult_latency "Multiplier Latency"; add_latency "Adder Latency"; conv_latency "Convert latency"; conjugated "Conjugate"; async "asynchronous operation"; pipelined_enable "enable pipeline"; multiplier_implementation "Multiplier implementation"
      mask help:
      | Multiplies two complex numbers using 4 multipliers and 2 adders.
      | Conjugation is optional.
      mask init: same as test_sys3/cmult
      settings: AttributesFormatString=|
      | 40_22 * 15_13 ==> 56_35
      | Truncate, Wrap
      | Latency=0
      mask TypeOptions quantization: Truncate | Round  (unbiased: +/- Inf) | Round  (unbiased: Even Values)
      mask TypeOptions overflow: Wrap | Saturate | Flag as error
      mask TypeOptions multiplier_implementation: behavioral HDL | standard core | embedded multiplier core
  msdft_comb : Subsystem  mask(msdft_comb){input_bitsize=10, fft_len=7, latency=0}
      mask prompts: fft_len "fft_len (2^?)"; latency "sub latency"
      mask init:
      | msdft_comb_init(gcb, ...
      |         'input_bitsize', input_bitsize, ...
      |         'fft_len', fft_len, ...
      |         'latency', latency);
      settings: AttributesFormatString=latency=0
  power{,1..31} (32 alike) : casper_library_misc/power  BitWidth=56  add_latency=2  mult_latency=3
  resonator : Subsystem  mask(msdft_res){fft_len=7, twid_bitsize=15, bin_number=0, input_bitsize=11, input_frac=9, res_bitsize=40, add_lat=0}
      mask prompts: fft_len "fft len(2^?)"; twid_bitsize "twid bitsize"; bin_number "bin number"; input_bitsize "input bitsize"; input_frac "input frac"; res_bitsize "out resonator size"
      mask init:
      | msdft_resonator_init(gcb, ...
      |                 'fft_len', fft_len, ...
      |                 'twid_bitsize', twid_bitsize, ...
      |                 'bin_number', bin_number, ...
      |                 'input_bitsize', input_bitsize, ...
      |                 'input_frac', input_frac, ...
      |                 'res_bitsize', res_bitsize, ...
      |                 'add_lat', add_lat);
      settings: AttributesFormatString=N=7, k=0
  resonator1 : Subsystem  mask(msdft_res){fft_len=7, twid_bitsize=15, bin_number=1, input_bitsize=11, input_frac=9, res_bitsize=40, add_lat=0}
      mask prompts: fft_len "fft len(2^?)"; twid_bitsize "twid bitsize"; bin_number "bin number"; input_bitsize "input bitsize"; input_frac "input frac"; res_bitsize "out resonator size"
      mask init: same as test_sys3/resonator
      settings: AttributesFormatString=N=7, k=1
  resonator10 : Subsystem  mask(msdft_res){fft_len=7, twid_bitsize=15, bin_number=10, input_bitsize=11, input_frac=9, res_bitsize=40, add_lat=0}
      mask prompts: fft_len "fft len(2^?)"; twid_bitsize "twid bitsize"; bin_number "bin number"; input_bitsize "input bitsize"; input_frac "input frac"; res_bitsize "out resonator size"
      mask init: same as test_sys3/resonator
      settings: AttributesFormatString=N=7, k=10
  resonator11 : Subsystem  mask(msdft_res){fft_len=7, twid_bitsize=15, bin_number=11, input_bitsize=11, input_frac=9, res_bitsize=40, add_lat=0}
      mask prompts: fft_len "fft len(2^?)"; twid_bitsize "twid bitsize"; bin_number "bin number"; input_bitsize "input bitsize"; input_frac "input frac"; res_bitsize "out resonator size"
      mask init: same as test_sys3/resonator
      settings: AttributesFormatString=N=7, k=11
  resonator12 : Subsystem  mask(msdft_res){fft_len=7, twid_bitsize=15, bin_number=12, input_bitsize=11, input_frac=9, res_bitsize=40, add_lat=0}
      mask prompts: fft_len "fft len(2^?)"; twid_bitsize "twid bitsize"; bin_number "bin number"; input_bitsize "input bitsize"; input_frac "input frac"; res_bitsize "out resonator size"
      mask init: same as test_sys3/resonator
      settings: AttributesFormatString=N=7, k=12
  resonator13 : Subsystem  mask(msdft_res){fft_len=7, twid_bitsize=15, bin_number=13, input_bitsize=11, input_frac=9, res_bitsize=40, add_lat=0}
      mask prompts: fft_len "fft len(2^?)"; twid_bitsize "twid bitsize"; bin_number "bin number"; input_bitsize "input bitsize"; input_frac "input frac"; res_bitsize "out resonator size"
      mask init: same as test_sys3/resonator
      settings: AttributesFormatString=N=7, k=13
  resonator14 : Subsystem  mask(msdft_res){fft_len=7, twid_bitsize=15, bin_number=31, input_bitsize=11, input_frac=9, res_bitsize=40, add_lat=0}
      mask prompts: fft_len "fft len(2^?)"; twid_bitsize "twid bitsize"; bin_number "bin number"; input_bitsize "input bitsize"; input_frac "input frac"; res_bitsize "out resonator size"
      mask init: same as test_sys3/resonator
      settings: AttributesFormatString=N=7, k=31
  resonator15 : Subsystem  mask(msdft_res){fft_len=7, twid_bitsize=15, bin_number=14, input_bitsize=11, input_frac=9, res_bitsize=40, add_lat=0}
      mask prompts: fft_len "fft len(2^?)"; twid_bitsize "twid bitsize"; bin_number "bin number"; input_bitsize "input bitsize"; input_frac "input frac"; res_bitsize "out resonator size"
      mask init: same as test_sys3/resonator
      settings: AttributesFormatString=N=7, k=14
  resonator16 : Subsystem  mask(msdft_res){fft_len=7, twid_bitsize=15, bin_number=15, input_bitsize=11, input_frac=9, res_bitsize=40, add_lat=0}
      mask prompts: fft_len "fft len(2^?)"; twid_bitsize "twid bitsize"; bin_number "bin number"; input_bitsize "input bitsize"; input_frac "input frac"; res_bitsize "out resonator size"
      mask init: same as test_sys3/resonator
      settings: AttributesFormatString=N=7, k=15
  resonator17 : Subsystem  mask(msdft_res){fft_len=7, twid_bitsize=15, bin_number=16, input_bitsize=11, input_frac=9, res_bitsize=40, add_lat=0}
      mask prompts: fft_len "fft len(2^?)"; twid_bitsize "twid bitsize"; bin_number "bin number"; input_bitsize "input bitsize"; input_frac "input frac"; res_bitsize "out resonator size"
      mask init: same as test_sys3/resonator
      settings: AttributesFormatString=N=7, k=16
  resonator18 : Subsystem  mask(msdft_res){fft_len=7, twid_bitsize=15, bin_number=17, input_bitsize=11, input_frac=9, res_bitsize=40, add_lat=0}
      mask prompts: fft_len "fft len(2^?)"; twid_bitsize "twid bitsize"; bin_number "bin number"; input_bitsize "input bitsize"; input_frac "input frac"; res_bitsize "out resonator size"
      mask init: same as test_sys3/resonator
      settings: AttributesFormatString=N=7, k=17
  resonator19 : Subsystem  mask(msdft_res){fft_len=7, twid_bitsize=15, bin_number=18, input_bitsize=11, input_frac=9, res_bitsize=40, add_lat=0}
      mask prompts: fft_len "fft len(2^?)"; twid_bitsize "twid bitsize"; bin_number "bin number"; input_bitsize "input bitsize"; input_frac "input frac"; res_bitsize "out resonator size"
      mask init: same as test_sys3/resonator
      settings: AttributesFormatString=N=7, k=18
  resonator2 : Subsystem  mask(msdft_res){fft_len=7, twid_bitsize=15, bin_number=2, input_bitsize=11, input_frac=9, res_bitsize=40, add_lat=0}
      mask prompts: fft_len "fft len(2^?)"; twid_bitsize "twid bitsize"; bin_number "bin number"; input_bitsize "input bitsize"; input_frac "input frac"; res_bitsize "out resonator size"
      mask init: same as test_sys3/resonator
      settings: AttributesFormatString=N=7, k=2
  resonator20 : Subsystem  mask(msdft_res){fft_len=7, twid_bitsize=15, bin_number=19, input_bitsize=11, input_frac=9, res_bitsize=40, add_lat=0}
      mask prompts: fft_len "fft len(2^?)"; twid_bitsize "twid bitsize"; bin_number "bin number"; input_bitsize "input bitsize"; input_frac "input frac"; res_bitsize "out resonator size"
      mask init: same as test_sys3/resonator
      settings: AttributesFormatString=N=7, k=19
  resonator21 : Subsystem  mask(msdft_res){fft_len=7, twid_bitsize=15, bin_number=20, input_bitsize=11, input_frac=9, res_bitsize=40, add_lat=0}
      mask prompts: fft_len "fft len(2^?)"; twid_bitsize "twid bitsize"; bin_number "bin number"; input_bitsize "input bitsize"; input_frac "input frac"; res_bitsize "out resonator size"
      mask init: same as test_sys3/resonator
      settings: AttributesFormatString=N=7, k=20
  resonator22 : Subsystem  mask(msdft_res){fft_len=7, twid_bitsize=15, bin_number=21, input_bitsize=11, input_frac=9, res_bitsize=40, add_lat=0}
      mask prompts: fft_len "fft len(2^?)"; twid_bitsize "twid bitsize"; bin_number "bin number"; input_bitsize "input bitsize"; input_frac "input frac"; res_bitsize "out resonator size"
      mask init: same as test_sys3/resonator
      settings: AttributesFormatString=N=7, k=21
  resonator23 : Subsystem  mask(msdft_res){fft_len=7, twid_bitsize=15, bin_number=22, input_bitsize=11, input_frac=9, res_bitsize=40, add_lat=0}
      mask prompts: fft_len "fft len(2^?)"; twid_bitsize "twid bitsize"; bin_number "bin number"; input_bitsize "input bitsize"; input_frac "input frac"; res_bitsize "out resonator size"
      mask init: same as test_sys3/resonator
      settings: AttributesFormatString=N=7, k=22
  resonator24 : Subsystem  mask(msdft_res){fft_len=7, twid_bitsize=15, bin_number=23, input_bitsize=11, input_frac=9, res_bitsize=40, add_lat=0}
      mask prompts: fft_len "fft len(2^?)"; twid_bitsize "twid bitsize"; bin_number "bin number"; input_bitsize "input bitsize"; input_frac "input frac"; res_bitsize "out resonator size"
      mask init: same as test_sys3/resonator
      settings: AttributesFormatString=N=7, k=23
  resonator25 : Subsystem  mask(msdft_res){fft_len=7, twid_bitsize=15, bin_number=24, input_bitsize=11, input_frac=9, res_bitsize=40, add_lat=0}
      mask prompts: fft_len "fft len(2^?)"; twid_bitsize "twid bitsize"; bin_number "bin number"; input_bitsize "input bitsize"; input_frac "input frac"; res_bitsize "out resonator size"
      mask init: same as test_sys3/resonator
      settings: AttributesFormatString=N=7, k=24
  resonator26 : Subsystem  mask(msdft_res){fft_len=7, twid_bitsize=15, bin_number=25, input_bitsize=11, input_frac=9, res_bitsize=40, add_lat=0}
      mask prompts: fft_len "fft len(2^?)"; twid_bitsize "twid bitsize"; bin_number "bin number"; input_bitsize "input bitsize"; input_frac "input frac"; res_bitsize "out resonator size"
      mask init: same as test_sys3/resonator
      settings: AttributesFormatString=N=7, k=25
  resonator27 : Subsystem  mask(msdft_res){fft_len=7, twid_bitsize=15, bin_number=26, input_bitsize=11, input_frac=9, res_bitsize=40, add_lat=0}
      mask prompts: fft_len "fft len(2^?)"; twid_bitsize "twid bitsize"; bin_number "bin number"; input_bitsize "input bitsize"; input_frac "input frac"; res_bitsize "out resonator size"
      mask init: same as test_sys3/resonator
      settings: AttributesFormatString=N=7, k=26
  resonator28 : Subsystem  mask(msdft_res){fft_len=7, twid_bitsize=15, bin_number=27, input_bitsize=11, input_frac=9, res_bitsize=40, add_lat=0}
      mask prompts: fft_len "fft len(2^?)"; twid_bitsize "twid bitsize"; bin_number "bin number"; input_bitsize "input bitsize"; input_frac "input frac"; res_bitsize "out resonator size"
      mask init: same as test_sys3/resonator
      settings: AttributesFormatString=N=7, k=27
  resonator29 : Subsystem  mask(msdft_res){fft_len=7, twid_bitsize=15, bin_number=28, input_bitsize=11, input_frac=9, res_bitsize=40, add_lat=0}
      mask prompts: fft_len "fft len(2^?)"; twid_bitsize "twid bitsize"; bin_number "bin number"; input_bitsize "input bitsize"; input_frac "input frac"; res_bitsize "out resonator size"
      mask init: same as test_sys3/resonator
      settings: AttributesFormatString=N=7, k=28
  resonator3 : Subsystem  mask(msdft_res){fft_len=7, twid_bitsize=15, bin_number=3, input_bitsize=11, input_frac=9, res_bitsize=40, add_lat=0}
      mask prompts: fft_len "fft len(2^?)"; twid_bitsize "twid bitsize"; bin_number "bin number"; input_bitsize "input bitsize"; input_frac "input frac"; res_bitsize "out resonator size"
      mask init: same as test_sys3/resonator
      settings: AttributesFormatString=N=7, k=3
  resonator30 : Subsystem  mask(msdft_res){fft_len=7, twid_bitsize=15, bin_number=29, input_bitsize=11, input_frac=9, res_bitsize=40, add_lat=0}
      mask prompts: fft_len "fft len(2^?)"; twid_bitsize "twid bitsize"; bin_number "bin number"; input_bitsize "input bitsize"; input_frac "input frac"; res_bitsize "out resonator size"
      mask init: same as test_sys3/resonator
      settings: AttributesFormatString=N=7, k=29
  resonator31 : Subsystem  mask(msdft_res){fft_len=7, twid_bitsize=15, bin_number=30, input_bitsize=11, input_frac=9, res_bitsize=40, add_lat=0}
      mask prompts: fft_len "fft len(2^?)"; twid_bitsize "twid bitsize"; bin_number "bin number"; input_bitsize "input bitsize"; input_frac "input frac"; res_bitsize "out resonator size"
      mask init: same as test_sys3/resonator
      settings: AttributesFormatString=N=7, k=30
  resonator4 : Subsystem  mask(msdft_res){fft_len=7, twid_bitsize=15, bin_number=4, input_bitsize=11, input_frac=9, res_bitsize=40, add_lat=0}
      mask prompts: fft_len "fft len(2^?)"; twid_bitsize "twid bitsize"; bin_number "bin number"; input_bitsize "input bitsize"; input_frac "input frac"; res_bitsize "out resonator size"
      mask init: same as test_sys3/resonator
      settings: AttributesFormatString=N=7, k=4
  resonator5 : Subsystem  mask(msdft_res){fft_len=7, twid_bitsize=15, bin_number=5, input_bitsize=11, input_frac=9, res_bitsize=40, add_lat=0}
      mask prompts: fft_len "fft len(2^?)"; twid_bitsize "twid bitsize"; bin_number "bin number"; input_bitsize "input bitsize"; input_frac "input frac"; res_bitsize "out resonator size"
      mask init: same as test_sys3/resonator
      settings: AttributesFormatString=N=7, k=5
  resonator6 : Subsystem  mask(msdft_res){fft_len=7, twid_bitsize=15, bin_number=6, input_bitsize=11, input_frac=9, res_bitsize=40, add_lat=0}
      mask prompts: fft_len "fft len(2^?)"; twid_bitsize "twid bitsize"; bin_number "bin number"; input_bitsize "input bitsize"; input_frac "input frac"; res_bitsize "out resonator size"
      mask init: same as test_sys3/resonator
      settings: AttributesFormatString=N=7, k=6
  resonator7 : Subsystem  mask(msdft_res){fft_len=7, twid_bitsize=15, bin_number=7, input_bitsize=11, input_frac=9, res_bitsize=40, add_lat=0}
      mask prompts: fft_len "fft len(2^?)"; twid_bitsize "twid bitsize"; bin_number "bin number"; input_bitsize "input bitsize"; input_frac "input frac"; res_bitsize "out resonator size"
      mask init: same as test_sys3/resonator
      settings: AttributesFormatString=N=7, k=7
  resonator8 : Subsystem  mask(msdft_res){fft_len=7, twid_bitsize=15, bin_number=8, input_bitsize=11, input_frac=9, res_bitsize=40, add_lat=0}
      mask prompts: fft_len "fft len(2^?)"; twid_bitsize "twid bitsize"; bin_number "bin number"; input_bitsize "input bitsize"; input_frac "input frac"; res_bitsize "out resonator size"
      mask init: same as test_sys3/resonator
      settings: AttributesFormatString=N=7, k=8
  resonator9 : Subsystem  mask(msdft_res){fft_len=7, twid_bitsize=15, bin_number=9, input_bitsize=11, input_frac=9, res_bitsize=40, add_lat=0}
      mask prompts: fft_len "fft len(2^?)"; twid_bitsize "twid bitsize"; bin_number "bin number"; input_bitsize "input bitsize"; input_frac "input frac"; res_bitsize "out resonator size"
      mask init: same as test_sys3/resonator
      settings: AttributesFormatString=N=7, k=9
  ri_to_c : casper_library_misc/ri_to_c
  wires:
  Constant1/1 -> Delay1/1, msdft_comb/2(rst)
  resonator/2(twidd) -> cmult/2(b)
  power/1 -> Reinterpret/1
  Gateway Out/1 -> To Workspace/1
  From Workspace/1 -> Gateway In/1
  resonator1/2(twidd) -> cmult1/2(b)
  power1/1 -> Reinterpret1/1
  Gateway Out1/1 -> To Workspace1/1
  resonator2/2(twidd) -> cmult2/2(b)
  power2/1 -> Reinterpret2/1
  Gateway Out2/1 -> To Workspace2/1
  resonator3/2(twidd) -> cmult3/2(b)
  power3/1 -> Reinterpret3/1
  Gateway Out3/1 -> To Workspace3/1
  resonator4/2(twidd) -> cmult4/2(b)
  power4/1 -> Reinterpret4/1
  Gateway Out4/1 -> To Workspace4/1
  resonator5/2(twidd) -> cmult5/2(b)
  power5/1 -> Reinterpret5/1
  Gateway Out5/1 -> To Workspace5/1
  resonator6/2(twidd) -> cmult6/2(b)
  power6/1 -> Reinterpret6/1
  Gateway Out6/1 -> To Workspace6/1
  resonator7/2(twidd) -> cmult7/2(b)
  power7/1 -> Reinterpret7/1
  Gateway Out7/1 -> To Workspace7/1
  resonator8/2(twidd) -> cmult8/2(b)
  power8/1 -> Reinterpret8/1
  Gateway Out8/1 -> To Workspace8/1
  resonator9/2(twidd) -> cmult9/2(b)
  power9/1 -> Reinterpret9/1
  Gateway Out9/1 -> To Workspace9/1
  resonator10/2(twidd) -> cmult10/2(b)
  power10/1 -> Reinterpret10/1
  Gateway Out10/1 -> To Workspace10/1
  msdft_comb/1(dout) -> resonator16/1(din), resonator13/1(din), resonator12/1(din), resonator11/1(din), resonator10/1(din), resonator9/1(din), resonator5/1(din), resonator4/1(din), resonator2/1(din), resonator1/1(din), c_to_ri/1, resonator/1(din), resonator3/1(din), resonator6/1(din), resonator7/1(din), resonator8/1(din), resonator15/1(din), resonator17/1(din), resonator18/1(din), resonator19/1(din), resonator21/1(din), resonator23/1(din), resonator24/1(din), resonator25/1(din), resonator27/1(din), resonator28/1(din), resonator29/1(din), resonator31/1(din), resonator14/1(din), resonator30/1(din), resonator26/1(din), resonator22/1(din), resonator20/1(din)
  Delay2/1 -> resonator17/2(sync), resonator21/2(sync), resonator31/2(sync), resonator14/2(sync), resonator30/2(sync), resonator29/2(sync), resonator28/2(sync), resonator27/2(sync), resonator26/2(sync), resonator25/2(sync), resonator24/2(sync), resonator23/2(sync), resonator22/2(sync), resonator20/2(sync), resonator19/2(sync), resonator18/2(sync), resonator16/2(sync), resonator15/2(sync), resonator13/2(sync), resonator12/2(sync), resonator11/2(sync), resonator10/2(sync), resonator9/2(sync), resonator6/2(sync), resonator5/2(sync), resonator4/2(sync), resonator3/2(sync), resonator2/2(sync), resonator1/2(sync), resonator/2(sync), resonator7/2(sync), resonator8/2(sync)
  Delay1/1 -> resonator15/3(rst), resonator18/3(rst), resonator25/3(rst), resonator28/3(rst), resonator29/3(rst), resonator30/3(rst), resonator14/3(rst), resonator31/3(rst), resonator27/3(rst), resonator26/3(rst), resonator24/3(rst), resonator23/3(rst), resonator22/3(rst), resonator21/3(rst), resonator20/3(rst), resonator19/3(rst), resonator17/3(rst), resonator16/3(rst), resonator13/3(rst), resonator12/3(rst), resonator11/3(rst), resonator10/3(rst), resonator9/3(rst), resonator8/3(rst), resonator6/3(rst), resonator5/3(rst), resonator4/3(rst), resonator3/3(rst), resonator2/3(rst), resonator1/3(rst), resonator/3(rst), resonator7/3(rst)
  resonator11/2(twidd) -> cmult11/2(b)
  power11/1 -> Reinterpret11/1
  Gateway Out11/1 -> To Workspace11/1
  resonator12/2(twidd) -> cmult12/2(b)
  power12/1 -> Reinterpret12/1
  Gateway Out12/1 -> To Workspace12/1
  resonator13/2(twidd) -> cmult13/2(b)
  power13/1 -> Reinterpret13/1
  Gateway Out13/1 -> To Workspace13/1
  power14/1 -> Reinterpret31/1
  Gateway Out14/1 -> To Workspace14/1
  resonator15/2(twidd) -> cmult14/2(b)
  power15/1 -> Reinterpret14/1
  Gateway Out15/1 -> To Workspace15/1
  resonator16/2(twidd) -> cmult15/2(b)
  power16/1 -> Reinterpret15/1
  Gateway Out16/1 -> To Workspace16/1
  resonator17/2(twidd) -> cmult16/2(b)
  power17/1 -> Reinterpret16/1
  Gateway Out17/1 -> To Workspace17/1
  resonator18/2(twidd) -> cmult17/2(b)
  power18/1 -> Reinterpret17/1
  Gateway Out18/1 -> To Workspace18/1
  resonator19/2(twidd) -> cmult18/2(b)
  power19/1 -> Reinterpret18/1
  Gateway Out19/1 -> To Workspace19/1
  resonator20/2(twidd) -> cmult19/2(b)
  power20/1 -> Reinterpret19/1
  Gateway Out20/1 -> To Workspace20/1
  resonator21/2(twidd) -> cmult20/2(b)
  power21/1 -> Reinterpret20/1
  Gateway Out21/1 -> To Workspace21/1
  resonator22/2(twidd) -> cmult21/2(b)
  power22/1 -> Reinterpret21/1
  Gateway Out22/1 -> To Workspace22/1
  resonator23/2(twidd) -> cmult22/2(b)
  power23/1 -> Reinterpret22/1
  Gateway Out23/1 -> To Workspace23/1
  power24/1 -> Reinterpret23/1
  Gateway Out24/1 -> To Workspace24/1
  power25/1 -> Reinterpret24/1
  Gateway Out25/1 -> To Workspace25/1
  power26/1 -> Reinterpret25/1
  Gateway Out26/1 -> To Workspace26/1
  power27/1 -> Reinterpret26/1
  Gateway Out27/1 -> To Workspace27/1
  power28/1 -> Reinterpret27/1
  Gateway Out28/1 -> To Workspace28/1
  power29/1 -> Reinterpret28/1
  Gateway Out29/1 -> To Workspace29/1
  power30/1 -> Reinterpret29/1
  Gateway Out30/1 -> To Workspace30/1
  power31/1 -> Reinterpret30/1
  Gateway Out31/1 -> To Workspace31/1
  Gateway In/1 -> [input], ri_to_c/1
  Constant/1 -> ri_to_c/2
  ri_to_c/1 -> msdft_comb/3(din)
  Constant2/1 -> Delay2/1, msdft_comb/1(sync)
  c_to_ri/1 -> Gateway Out32/1
  c_to_ri/2 -> Gateway Out33/1
  Gateway Out32/1 -> To Workspace32/1
  Gateway Out33/1 -> To Workspace33/1
  Reinterpret/1 -> Gateway Out/1
  Reinterpret1/1 -> Gateway Out1/1
  Reinterpret2/1 -> Gateway Out2/1
  Reinterpret3/1 -> Gateway Out3/1
  Reinterpret4/1 -> Gateway Out4/1
  Reinterpret5/1 -> Gateway Out5/1
  Reinterpret6/1 -> Gateway Out6/1
  Reinterpret7/1 -> Gateway Out7/1
  Reinterpret8/1 -> Gateway Out8/1
  Reinterpret9/1 -> Gateway Out9/1
  Reinterpret10/1 -> Gateway Out10/1
  Reinterpret11/1 -> Gateway Out11/1
  Reinterpret12/1 -> Gateway Out12/1
  Reinterpret13/1 -> Gateway Out13/1
  Reinterpret14/1 -> Gateway Out15/1
  Reinterpret15/1 -> Gateway Out16/1
  Reinterpret16/1 -> Gateway Out17/1
  Reinterpret17/1 -> Gateway Out18/1
  Reinterpret18/1 -> Gateway Out19/1
  Reinterpret19/1 -> Gateway Out20/1
  Reinterpret20/1 -> Gateway Out21/1
  Reinterpret21/1 -> Gateway Out22/1
  Reinterpret22/1 -> Gateway Out23/1
  Reinterpret23/1 -> Gateway Out24/1
  Reinterpret24/1 -> Gateway Out25/1
  Reinterpret25/1 -> Gateway Out26/1
  Reinterpret26/1 -> Gateway Out27/1
  Reinterpret27/1 -> Gateway Out28/1
  Reinterpret28/1 -> Gateway Out29/1
  Reinterpret29/1 -> Gateway Out30/1
  Reinterpret30/1 -> Gateway Out31/1
  Reinterpret31/1 -> Gateway Out14/1
  resonator/1(Out1) -> cmult/1(a)
  resonator1/1(Out1) -> cmult1/1(a)
  resonator2/1(Out1) -> cmult2/1(a)
  resonator3/1(Out1) -> cmult3/1(a)
  resonator4/1(Out1) -> cmult4/1(a)
  resonator5/1(Out1) -> cmult5/1(a)
  resonator6/1(Out1) -> cmult6/1(a)
  resonator7/1(Out1) -> cmult7/1(a)
  resonator8/1(Out1) -> cmult8/1(a)
  resonator9/1(Out1) -> cmult9/1(a)
  resonator10/1(Out1) -> cmult10/1(a)
  resonator11/1(Out1) -> cmult11/1(a)
  resonator12/1(Out1) -> cmult12/1(a)
  resonator13/1(Out1) -> cmult13/1(a)
  resonator15/1(Out1) -> cmult14/1(a)
  resonator16/1(Out1) -> cmult15/1(a)
  resonator17/1(Out1) -> cmult16/1(a)
  resonator18/1(Out1) -> cmult17/1(a)
  resonator19/1(Out1) -> cmult18/1(a)
  resonator20/1(Out1) -> cmult19/1(a)
  resonator21/1(Out1) -> cmult20/1(a)
  resonator22/1(Out1) -> cmult21/1(a)
  resonator23/1(Out1) -> cmult22/1(a)
  resonator24/2(twidd) -> cmult23/2(b)
  resonator24/1(Out1) -> cmult23/1(a)
  resonator25/1(Out1) -> cmult24/1(a)
  resonator25/2(twidd) -> cmult24/2(b)
  resonator26/2(twidd) -> cmult25/2(b)
  resonator26/1(Out1) -> cmult25/1(a)
  resonator27/2(twidd) -> cmult26/2(b)
  resonator27/1(Out1) -> cmult26/1(a)
  resonator28/2(twidd) -> cmult27/2(b)
  resonator28/1(Out1) -> cmult27/1(a)
  resonator29/2(twidd) -> cmult28/2(b)
  resonator29/1(Out1) -> cmult28/1(a)
  resonator30/2(twidd) -> cmult29/2(b)
  resonator30/1(Out1) -> cmult29/1(a)
  resonator31/2(twidd) -> cmult30/2(b)
  resonator31/1(Out1) -> cmult30/1(a)
  resonator14/1(Out1) -> cmult31/1(a)
  resonator14/2(twidd) -> cmult31/2(b)
  cmult/1(ab) -> power/1
  cmult1/1(ab) -> power1/1
  cmult2/1(ab) -> power2/1
  cmult3/1(ab) -> power3/1
  cmult4/1(ab) -> power4/1
  cmult5/1(ab) -> power5/1
  cmult6/1(ab) -> power6/1
  cmult7/1(ab) -> power7/1
  cmult8/1(ab) -> power8/1
  cmult9/1(ab) -> power9/1
  cmult10/1(ab) -> power10/1
  cmult11/1(ab) -> power11/1
  cmult12/1(ab) -> power12/1
  cmult13/1(ab) -> power13/1
  cmult14/1(ab) -> power15/1
  cmult15/1(ab) -> power16/1
  cmult17/1(ab) -> power18/1
  cmult18/1(ab) -> power19/1
  cmult19/1(ab) -> power20/1
  cmult20/1(ab) -> power21/1
  cmult21/1(ab) -> power22/1
  cmult22/1(ab) -> power23/1
  cmult23/1(ab) -> power24/1
  cmult24/1(ab) -> power25/1
  cmult25/1(ab) -> power26/1
  cmult26/1(ab) -> power27/1
  cmult27/1(ab) -> power28/1
  cmult28/1(ab) -> power29/1
  cmult29/1(ab) -> power30/1
  cmult30/1(ab) -> power31/1
  cmult31/1(ab) -> power14/1
  cmult16/1(ab) -> power17/1
